simulink model "control_UAV"  (R2026a)
settings: Solver=VariableStepAuto  StopTime=30
values from neighbouring files (symbols this model uses):
  b = P.rotor.b    [Inicializacion.m]
  chen_a = 35    [Inicializacion.m]
  chen_b = 3    [Inicializacion.m]
  chen_c = 28    [Inicializacion.m]
  chen_center_z = 30    [Inicializacion.m]
  chen_scale_x = 30    [Inicializacion.m]
  chen_scale_y = 35    [Inicializacion.m]
  chen_scale_z = 30    [Inicializacion.m]
  d = P.rotor.d    [Inicializacion.m]
  g = P.g    [Inicializacion.m]
  Jr = P.Jr    [Inicializacion.m]
  Jxx = P.Jxx    [Inicializacion.m]
  Jyy = P.Jyy    [Inicializacion.m]
  Jzz = P.Jzz    [Inicializacion.m]
  kdphi = K.phi.Kd    [Inicializacion.m]
  kdpsi = K.psi.Kd    [Inicializacion.m]
  kdtheta = K.theta.Kd    [Inicializacion.m]
  kDx = P.aero.kDx    [Inicializacion.m]
  kdx = K.x.Kd    [Inicializacion.m]
  kDy = P.aero.kDy    [Inicializacion.m]
  kdy = K.y.Kd    [Inicializacion.m]
  kDz = P.aero.kDz    [Inicializacion.m]
  kdz = K.zAccel.Kd    [Inicializacion.m]
  kfax = P.kfax    [Inicializacion.m]
  kfay = P.kfay    [Inicializacion.m]
  kfaz = P.kfaz    [Inicializacion.m]
  kftx = P.kftx    [Inicializacion.m]
  kfty = P.kfty    [Inicializacion.m]
  kftz = P.kftz    [Inicializacion.m]
  kiphi = K.phi.Ki    [Inicializacion.m]
  kipsi = K.psi.Ki    [Inicializacion.m]
  kitheta = K.theta.Ki    [Inicializacion.m]
  kix = K.x.Ki    [Inicializacion.m]
  kiy = K.y.Ki    [Inicializacion.m]
  kiz = K.zAccel.Ki    [Inicializacion.m]
  kpphi = K.phi.Kp    [Inicializacion.m]
  kppsi = K.psi.Kp    [Inicializacion.m]
  kptheta = K.theta.Kp    [Inicializacion.m]
  kpx = K.x.Kp    [Inicializacion.m]
  kpy = K.y.Kp    [Inicializacion.m]
  kpz = K.zAccel.Kp    [Inicializacion.m]
  l = P.armLength    [Inicializacion.m]
  m = P.mass    [Inicializacion.m]
  omega_max = P.rotor.omegaMax    [Inicializacion.m]
  tau_motor = 0.05    [Inicializacion.m]
  Thover = K.Thover    [Inicializacion.m]
  Vw_max = P.aero.windSpeedMax    [Inicializacion.m]
undefined symbols (not defined in the file or in its folder): magnitude
settings Model: Creator=d1vad_l3gna  LastModifiedBy=D1vad L3gna

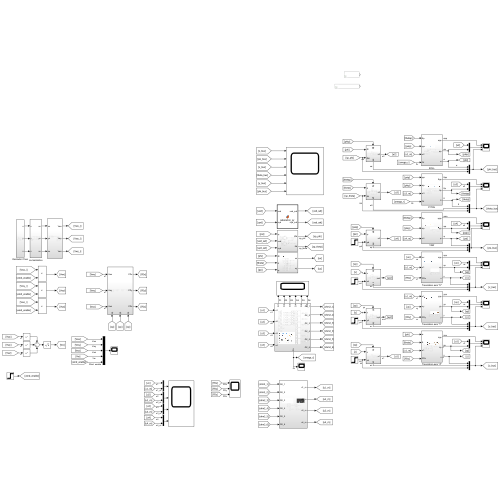
[thumbnail: Simulink's stored preview of the top-level diagram]
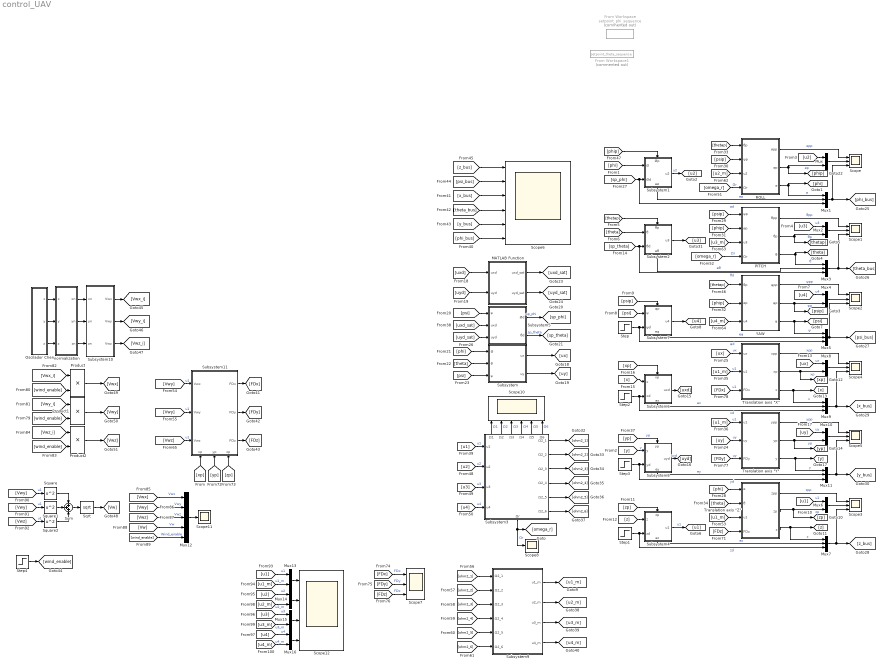
== system control_UAV ==
  From Workspace : FromWorkspace  Commented=on  VariableName=setpoint_phi_sequence  Interpolate=off  OutputAfterFinalValue=Holding final value
  From Workspace1 : FromWorkspace  Commented=on  VariableName=setpoint_theta_sequence  Interpolate=off  OutputAfterFinalValue=Holding final value
  MATLAB Function : MATLAB Function  TreatAsAtomicUnit=on
  Mux{,2,4,6,8,10,13..16} (10 alike) : Mux  Inputs=2
  Mux{1,3,5,7,9,11} (6 alike) : Mux  Inputs=3
  Mux12 : Mux  Inputs=5
  Oscilador Chen : Subsystem
  PITCH : Subsystem
  Product : Product
  Product1 : Product
  Product2 : Product
  ROLL : Subsystem
  Scope{,1..5,7} (7 alike) : Scope  NumInputPorts=3
      Scope settings: ActiveDisplayYMinimum=-134.04297196202708  ActiveDisplayYMaximum=108.05186605238116
      Scope1 settings: ActiveDisplayYMinimum=-2.6964368971416346  ActiveDisplayYMaximum=2.3091901291988428
      Scope2 settings: ActiveDisplayYMinimum=-20.085778959266992  ActiveDisplayYMaximum=163.07055659378912  DataLoggingVariableName=ScopeData2
      Scope3 settings: ActiveDisplayYMinimum=-60.018912358895363  ActiveDisplayYMaximum=169.44654581765505  DataLoggingVariableName=ScopeData3
      Scope4 settings: ActiveDisplayYMinimum=-60.018912358895363  ActiveDisplayYMaximum=169.44654581765505  DataLoggingVariableName=ScopeData4
      Scope5 settings: ActiveDisplayYMinimum=-4.0823822518726  ActiveDisplayYMaximum=2.5647555738372825  DataLoggingVariableName=ScopeData5
      Scope7 settings: ActiveDisplayString=3  ActiveDisplayYMinimum=-1.1101406632308159  ActiveDisplayYMaximum=0.27802164773982191  DataLoggingVariableName=ScopeData7
  Scope10 : Scope  NumInputPorts=6
      settings: ActiveDisplayYMinimum=-90.652821559527951  ActiveDisplayYMaximum=815.8753940357517  DataLoggingVariableName=ScopeData10
  Scope11 : Scope
      settings: ActiveDisplayYMinimum=-7.1247044664866621  ActiveDisplayYMaximum=8.6160020821192056  DataLoggingVariableName=ScopeData11
  Scope12 : Scope  NumInputPorts=4
      settings: ActiveDisplayYMinimum=-56.813279862399021  ActiveDisplayYMaximum=511.31951876159133  DataLoggingVariableName=ScopeData12
  Scope6 : Scope  NumInputPorts=6
      settings: ActiveDisplayYMinimum=-0.7400477310754251  ActiveDisplayYMaximum=5.6591974559880578  DataLoggingVariableName=ScopeData6
  Scope8 : Scope
      settings: ActiveDisplayYMinimum=-4.4408920985006262E-15  ActiveDisplayYMaximum=4.4408920985006262E-15  DataLoggingVariableName=ScopeData8
  Sqrt : Sqrt
  Square : Math  Operator=square
  Square1 : Math  Operator=square
  Square2 : Math  Operator=square
  Step : Step  Time=0  FinalValue=0  SampleTime=0
  Step1 : Step  FinalValue=5  SampleTime=0
  Step2 : Step  Time=4  FinalValue=5  SampleTime=0
  Step3 : Step  Time=0  FinalValue=0  SampleTime=0
  Step4 : Step  Time=9  SampleTime=0
  Subsystem : Subsystem
  Subsystem1 : Subsystem
      settings: PortSchema="{\"entries\":[{\"content\":{\"sides\":[{\"content\":{\"connectorIds\":[\"In1\",\"In2\"]},\"type\":\"ConnectorPlacement.EquallySpacedRectSide\",\"uuid\":\"d3a3a6fe-31b6-42e8-8951-59acef78037d\"},{\"content\":{\"connectorIds\":[\"Out1\"],\"side\":\"RIGHT\"},\"type\":\"ConnectorPlacement.EquallySpacedRectSide\",\"uuid\":\"98a273af-9231-4eb5-99d8-49a6c653f3f8\"},{\"content\":{\"connectorIds\":[\"In3\"],\"side\":\"TOP\"},\"type\":\"ConnectorPlacement.EquallySpacedRectSide\",\"uuid\":\"3e4d54af-1b05-4072-bd7d-c924a9f6a300\"},{\"content\":{\"connectorIds\":[\"Out2\"],\"side\":\"BOTTOM\"},\"type\":\"ConnectorPlacement.EquallySpacedRectSide\",\"uuid\":\"dbda693a-fe86-48a0-894d-0bd0198370e6\"}]},\"type\":\"ConnectorPlacement.EquallySpacedConnector\",\"uuid\":\"caea40f7-b591-4aba-8407-638933b38774\"}],\"packageUris\":[\"http://schema.mathworks.com/mf0/Connector/R2020b\"],\"version\":\"1.0\"}"
  Subsystem10 : Subsystem
  Subsystem11 : Subsystem
      settings: PortSchema="{\"entries\":[{\"content\":{\"sides\":[{\"content\":{\"connectorIds\":[\"In1\",\"In2\",\"In3\"]},\"type\":\"ConnectorPlacement.EquallySpacedRectSide\",\"uuid\":\"354ce72d-1d6c-4cc8-9e91-463c07f034cd\"},{\"content\":{\"connectorIds\":[\"Out1\",\"Out2\",\"Out3\"],\"side\":\"RIGHT\"},\"type\":\"ConnectorPlacement.EquallySpacedRectSide\",\"uuid\":\"d4bbd9c4-471b-4074-a3af-0e8a4cf51752\"},{\"content\":{\"side\":\"TOP\"},\"type\":\"ConnectorPlacement.EquallySpacedRectSide\",\"uuid\":\"5e614824-097c-4c07-9e45-0c4f9bbdd2e4\"},{\"content\":{\"connectorIds\":[\"In4\",\"In5\",\"In6\"],\"side\":\"BOTTOM\"},\"type\":\"ConnectorPlacement.EquallySpacedRectSide\",\"uuid\":\"b8e7f3a6-70ea-469a-9568-8fe2ed1a39af\"}]},\"type\":\"ConnectorPlacement.EquallySpacedConnector\",\"uuid\":\"e757125c-b99d-4f23-b824-7aca730001ba\"}],\"packageUris\":[\"http://schema.mathworks.com/mf0/Connector/R2020b\"],\"version\":\"1.0\"}"
  Subsystem2 : Subsystem
      settings: PortSchema="{\"entries\":[{\"content\":{\"sides\":[{\"content\":{\"connectorIds\":[\"In1\",\"In2\"]},\"type\":\"ConnectorPlacement.EquallySpacedRectSide\",\"uuid\":\"c42bea5d-3df1-43f4-8461-fc0f8e0dbc4c\"},{\"content\":{\"connectorIds\":[\"Out1\"],\"side\":\"RIGHT\"},\"type\":\"ConnectorPlacement.EquallySpacedRectSide\",\"uuid\":\"72025c3e-c054-42d9-8613-22244a708765\"},{\"content\":{\"connectorIds\":[\"In3\"],\"side\":\"TOP\"},\"type\":\"ConnectorPlacement.EquallySpacedRectSide\",\"uuid\":\"4b6680ac-412c-41ad-b127-e39dee57a48b\"},{\"content\":{\"connectorIds\":[\"Out2\"],\"side\":\"BOTTOM\"},\"type\":\"ConnectorPlacement.EquallySpacedRectSide\",\"uuid\":\"172eadf6-2acd-43c4-907f-43e59ecf9406\"}]},\"type\":\"ConnectorPlacement.EquallySpacedConnector\",\"uuid\":\"ee6badca-de14-4676-af90-b761200effe4\"}],\"packageUris\":[\"http://schema.mathworks.com/mf0/Connector/R2020b\"],\"version\":\"1.0\"}"
  Subsystem3 : Subsystem
      settings: PortSchema="{\"entries\":[{\"content\":{\"sides\":[{\"content\":{\"connectorIds\":[\"In1\",\"In2\",\"In3\",\"In4\"]},\"type\":\"ConnectorPlacement.EquallySpacedRectSide\",\"uuid\":\"bbf73f2c-001a-4d28-bdc9-6d66d68f2ea4\"},{\"content\":{\"connectorIds\":[\"Out1\",\"Out2\",\"Out3\",\"Out4\",\"Out5\",\"Out6\"],\"side\":\"RIGHT\"},\"type\":\"ConnectorPlacement.EquallySpacedRectSide\",\"uuid\":\"2f04f957-8e88-4bc3-9b02-53fc0fb1d7f8\"},{\"content\":{\"connectorIds\":[\"Out8\",\"Out9\",\"Out10\",\"Out11\",\"Out12\",\"Out13\"],\"side\":\"TOP\"},\"type\":\"ConnectorPlacement.EquallySpacedRectSide\",\"uuid\":\"66771ef2-ad1a-4f4f-bfbc-325ca576d4d7\"},{\"content\":{\"connectorIds\":[\"Out7\"],\"side\":\"BOTTOM\"},\"type\":\"ConnectorPlacement.EquallySpacedRectSide\",\"uuid\":\"4f342048-b513-46d4-854a-b011df012f9d\"}]},\"type\":\"ConnectorPlacement.EquallySpacedConnector\",\"uuid\":\"5b7006c4-ee2f-4b2d-a5a4-3391366b57a8\"}],\"packageUris\":[\"http://schema.mathworks.com/mf0/Connector/R2020b\"],\"version\":\"1.0\"}"
  Subsystem4 : Subsystem
      settings: PortSchema="{\"entries\":[{\"content\":{\"sides\":[{\"content\":{\"connectorIds\":[\"In1\",\"In2\"]},\"type\":\"ConnectorPlacement.EquallySpacedRectSide\",\"uuid\":\"05b9bfb1-b25d-4f19-883a-8c73fb6ccdf1\"},{\"content\":{\"connectorIds\":[\"Out1\"],\"side\":\"RIGHT\"},\"type\":\"ConnectorPlacement.EquallySpacedRectSide\",\"uuid\":\"b5ec7534-1bb3-4079-b442-bebab7b7e6ff\"},{\"content\":{\"connectorIds\":[\"In3\"],\"side\":\"TOP\"},\"type\":\"ConnectorPlacement.EquallySpacedRectSide\",\"uuid\":\"45979954-0dce-4b5e-a8a1-be246f039e3e\"},{\"content\":{\"connectorIds\":[\"Out2\"],\"side\":\"BOTTOM\"},\"type\":\"ConnectorPlacement.EquallySpacedRectSide\",\"uuid\":\"2779124c-2f03-4275-9de9-8b69c4e3182f\"}]},\"type\":\"ConnectorPlacement.EquallySpacedConnector\",\"uuid\":\"2b80c90b-fdf2-4625-bada-2e722c12cb75\"}],\"packageUris\":[\"http://schema.mathworks.com/mf0/Connector/R2020b\"],\"version\":\"1.0\"}"
  Subsystem5 : Subsystem
  Subsystem6 : Subsystem
      settings: PortSchema="{\"entries\":[{\"content\":{\"sides\":[{\"content\":{\"connectorIds\":[\"In1\",\"In2\"]},\"type\":\"ConnectorPlacement.EquallySpacedRectSide\",\"uuid\":\"d3a3a6fe-31b6-42e8-8951-59acef78037d\"},{\"content\":{\"connectorIds\":[\"Out1\"],\"side\":\"RIGHT\"},\"type\":\"ConnectorPlacement.EquallySpacedRectSide\",\"uuid\":\"98a273af-9231-4eb5-99d8-49a6c653f3f8\"},{\"content\":{\"connectorIds\":[\"In3\"],\"side\":\"TOP\"},\"type\":\"ConnectorPlacement.EquallySpacedRectSide\",\"uuid\":\"3e4d54af-1b05-4072-bd7d-c924a9f6a300\"},{\"content\":{\"connectorIds\":[\"Out2\"],\"side\":\"BOTTOM\"},\"type\":\"ConnectorPlacement.EquallySpacedRectSide\",\"uuid\":\"04a05dfd-3838-43e0-9a0f-9dddf1e0efcf\"}]},\"type\":\"ConnectorPlacement.EquallySpacedConnector\",\"uuid\":\"caea40f7-b591-4aba-8407-638933b38774\"}],\"packageUris\":[\"http://schema.mathworks.com/mf0/Connector/R2020b\"],\"version\":\"1.0\"}"
  Subsystem7 : Subsystem
      settings: PortSchema="{\"entries\":[{\"content\":{\"sides\":[{\"content\":{\"connectorIds\":[\"In1\",\"In2\"]},\"type\":\"ConnectorPlacement.EquallySpacedRectSide\",\"uuid\":\"75bf6914-bd39-4ffb-9926-3e582ee76d2e\"},{\"content\":{\"connectorIds\":[\"Out1\"],\"side\":\"RIGHT\"},\"type\":\"ConnectorPlacement.EquallySpacedRectSide\",\"uuid\":\"c513c889-9702-4896-9634-182684fb2270\"},{\"content\":{\"connectorIds\":[\"In3\"],\"side\":\"TOP\"},\"type\":\"ConnectorPlacement.EquallySpacedRectSide\",\"uuid\":\"615aeb91-fdc7-410e-8ef1-be935f8f6065\"},{\"content\":{\"connectorIds\":[\"Out2\"],\"side\":\"BOTTOM\"},\"type\":\"ConnectorPlacement.EquallySpacedRectSide\",\"uuid\":\"e306c6e8-76f5-43f1-b56c-f57f2096c31d\"}]},\"type\":\"ConnectorPlacement.EquallySpacedConnector\",\"uuid\":\"5b277172-4ad9-4051-981d-00b9cba435ce\"}],\"packageUris\":[\"http://schema.mathworks.com/mf0/Connector/R2020b\"],\"version\":\"1.0\"}"
  Subsystem8 : Subsystem
      settings: PortSchema="{\"entries\":[{\"content\":{\"sides\":[{\"content\":{\"connectorIds\":[\"In1\",\"In2\"]},\"type\":\"ConnectorPlacement.EquallySpacedRectSide\",\"uuid\":\"d3a3a6fe-31b6-42e8-8951-59acef78037d\"},{\"content\":{\"connectorIds\":[\"Out1\"],\"side\":\"RIGHT\"},\"type\":\"ConnectorPlacement.EquallySpacedRectSide\",\"uuid\":\"98a273af-9231-4eb5-99d8-49a6c653f3f8\"},{\"content\":{\"connectorIds\":[\"In3\"],\"side\":\"TOP\"},\"type\":\"ConnectorPlacement.EquallySpacedRectSide\",\"uuid\":\"3e4d54af-1b05-4072-bd7d-c924a9f6a300\"},{\"content\":{\"connectorIds\":[\"Out2\"],\"side\":\"BOTTOM\"},\"type\":\"ConnectorPlacement.EquallySpacedRectSide\",\"uuid\":\"3f53bca7-61ef-434d-b07d-c6d7aec8d75b\"}]},\"type\":\"ConnectorPlacement.EquallySpacedConnector\",\"uuid\":\"caea40f7-b591-4aba-8407-638933b38774\"}],\"packageUris\":[\"http://schema.mathworks.com/mf0/Connector/R2020b\"],\"version\":\"1.0\"}"
  Subsystem9 : Subsystem
  Sum : Sum  Inputs=+++
  "Translation axis \"X\"" : Subsystem
  "Translation axis \"Y\"" : Subsystem
  "Translation axis \"Z\"" : Subsystem
  YAW : Subsystem
  normalization : Subsystem
  wires:
  Subsystem1/1(u2) -> [u2]  "u2"
  [sp_phi] -> Mux1/3, Subsystem1/2(Ød)  "ød"
  Mux1/1 -> [phi_bus], Scope/3
  Mux/1 -> Scope/2
  [phi] -> Subsystem1/1(Ø)
  ROLL/1(øpp) -> Scope/1  "øpp"
  ROLL/2(øp) -> Mux/2, [phip]  "øp"
  ROLL/3(ø) -> [phi], Mux1/1  "ø"
  Subsystem1/2(eø) -> Mux1/2  "eø"
  Mux2/1 -> Scope1/2
  [sp_theta] -> Mux3/3, Subsystem2/2(θd)  "θd"
  PITCH/3(θ) -> [theta], Mux3/1  "θ"
  Subsystem2/2(eθ) -> Mux3/2  "eθ"
  Mux3/1 -> Scope1/3, [theta_bus]
  [thetap] -> Subsystem2/3(θp)
  PITCH/2(θp) -> Mux2/2, [thetap]  "θp"
  PITCH/1(θpp) -> Scope1/1  "θpp"
  [thetap] -> YAW/1(θp)
  YAW/1(ψpp) -> Scope2/1  "ψpp"
  YAW/2(ψp) -> [psip], Mux4/2  "ψp"
  Subsystem7/1(u4) -> [u4]
  Step/1 -> Mux5/3, Subsystem7/2(ψd)  "ψd"
  [u4] -> Mux4/1  "u4"
  Mux4/1 -> Scope2/2
  Mux5/1 -> Scope2/3, [psi_bus]
  YAW/3(ψ) -> Mux5/1, [psi]  "ψ"
  [psi] -> Subsystem7/1(ψ)
  [psip] -> Subsystem7/3(ψp)
  Subsystem7/2(eψ) -> Mux5/2  "eψ"
  [phi] -> "Translation axis \"Z\""/1(ø)
  [theta] -> "Translation axis \"Z\""/2(θ)
  Subsystem4/1(u1) -> [u1]  "u1"
  [u1] -> Mux6/1  "u1"
  "Translation axis \"Z\""/2(zp) -> [zp], Mux6/2  "zp"
  Step1/1 -> Mux7/3, Subsystem4/2(zd)  "zd"
  "Translation axis \"Z\""/3(z) -> Mux7/1, [z]  "z"
  Subsystem4/2(ez) -> Mux7/2  "ez"
  [zp] -> Subsystem4/3(zp)
  [z] -> Subsystem4/1(z)
  Mux6/1 -> Scope3/2
  Mux7/1 -> [z_bus], Scope3/3
  "Translation axis \"Z\""/1(zpp) -> Scope3/1  "zpp"
  Step2/1 -> Mux9/3, Subsystem6/2(xd)  "xd"
  [ux] -> Mux8/1  "ux"
  Mux8/1 -> Scope4/2
  "Translation axis \"X\""/1(xpp) -> Scope4/1  "xpp"
  "Translation axis \"X\""/2(xp) -> [xp], Mux8/2  "xp"
  "Translation axis \"X\""/3(x) -> Mux9/1, [x]  "x"
  [xp] -> Subsystem6/3(xp)
  [x] -> Subsystem6/1(x)
  Subsystem6/2(ex) -> Mux9/2  "ex"
  Mux9/1 -> [x_bus], Scope4/3
  Subsystem6/1(uxd) -> [uxd]
  Subsystem8/1(uyd) -> [uyd]  "uyd"
  Step3/1 -> Mux11/3, Subsystem8/2(yd)  "yd"
  Mux10/1 -> Scope5/2
  "Translation axis \"Y\""/1(ypp) -> Scope5/1  "ypp"
  [uy] -> Mux10/1  "uy"
  "Translation axis \"Y\""/2(yp) -> Mux10/2, [yp]  "yp"
  "Translation axis \"Y\""/3(y) -> Mux11/1, [y]  "y"
  Mux11/1 -> [y_bus], Scope5/3
  Subsystem8/2(ey) -> Mux11/2  "ey"
  [phi] -> Subsystem/1(Ø)
  [theta] -> Subsystem/2(θ)
  [psi] -> Subsystem/3(ψ)
  Subsystem/1(ux) -> [ux]
  Subsystem/2(uy) -> [uy]
  [uy] -> "Translation axis \"Y\""/2(uy)  "uy"
  [ux] -> "Translation axis \"X\""/1(ux)  "ux"
  Subsystem5/1(Ød) -> [sp_phi]  "sp_phi"
  Subsystem5/2(θd) -> [sp_theta]  "sp_theta"
  [u1_m] -> "Translation axis \"X\""/2(u1)  "u1"
  [u1_m] -> "Translation axis \"Y\""/1(u1)  "u1"
  [psi] -> Subsystem5/1(ψ)
  [uxd] -> MATLAB Function/1(uxd)
  [uyd] -> MATLAB Function/2(uyd)
  MATLAB Function/1(uxd_sat) -> [uxd_sat]
  MATLAB Function/2(uyd_sat) -> [uyd_sat]
  [uxd_sat] -> Subsystem5/2(uxd)
  [uyd_sat] -> Subsystem5/3(uyd)
  [z_bus] -> Scope6/1
  [psi_bus] -> Scope6/2
  [x_bus] -> Scope6/3
  [theta_bus] -> Scope6/4
  [y_bus] -> Scope6/5
  [phi_bus] -> Scope6/6
  [thetap] -> ROLL/1(θp)
  [psip] -> PITCH/1(ψp)
  [phip] -> PITCH/2(øp)
  [phip] -> YAW/2(øp)
  [yp] -> Subsystem8/3(yp)  "yp"
  [y] -> Subsystem8/1(y)  "y"
  [phip] -> Subsystem1/3(Øp)
  [theta] -> Subsystem2/1(θ)
  [u2] -> Mux/1
  [u3] -> Mux2/1  "u3"
  Subsystem2/1(u3) -> [u3]
  [psip] -> ROLL/2(ψp)
  [u1] -> Subsystem3/1(u1)  "u1"
  [u2] -> Subsystem3/2(u2)  "u2"
  [u3] -> Subsystem3/3(u3)  "u3"
  [u4] -> Subsystem3/4(u4)  "u4"
  Subsystem3/7(Ωr) -> [omega_r], Scope8/1  "Ωr"
  [omega_r] -> ROLL/4(Ωr)  "Ωr"
  [omega_r] -> PITCH/4(Ωr)  "Ωr"
  [u1_m] -> "Translation axis \"Z\""/3(u1)
  Subsystem3/2(Ω2_2) -> [ohm2_2]
  Subsystem3/3(Ω2_3) -> [ohm2_3]
  Subsystem3/4(Ω2_4) -> [ohm2_4]
  Subsystem3/6(Ω2_6) -> [ohm2_6]
  Subsystem3/8(Ω1) -> Scope10/1  "Ω1"
  Subsystem3/9(Ω2) -> Scope10/2  "Ω2"
  Subsystem3/10(Ω3) -> Scope10/3  "Ω3"
  Subsystem3/11(Ω4) -> Scope10/4  "Ω4"
  Subsystem3/12(Ω5) -> Scope10/5  "Ω5"
  Subsystem3/13(Ω6) -> Scope10/6  "Ω6"
  [ohm2_1] -> Subsystem9/1(Ω2_1)
  [ohm2_2] -> Subsystem9/2(Ω2_2)
  [ohm2_3] -> Subsystem9/3(Ω2_3)
  [ohm2_4] -> Subsystem9/4(Ω2_4)
  [ohm2_5] -> Subsystem9/5(Ω2_5)
  [ohm2_6] -> Subsystem9/6(Ω2_6)
  Subsystem9/1(u1_m) -> [u1_m]
  Subsystem9/2(u2_m) -> [u2_m]
  Subsystem9/3(u3_m) -> [u3_m]
  Subsystem9/4(u4_m) -> [u4_m]
  [u2_m] -> ROLL/3(u2)
  [u3_m] -> PITCH/3(u3)
  [u4_m] -> YAW/3(u4)
  Subsystem3/1(Ω2_1) -> [ohm2_1]
  Subsystem3/5(Ω2_5) -> [ohm2_5]
  Oscilador Chen/1(x) -> normalization/1(x)
  Oscilador Chen/2(y) -> normalization/2(y)
  Oscilador Chen/3(z) -> normalization/3(z)
  normalization/1(xn) -> Subsystem10/1(xn)
  normalization/2(yn) -> Subsystem10/2(yn)
  normalization/3(zn) -> Subsystem10/3(zn)
  [FDz] -> "Translation axis \"Z\""/4(FDz)
  [xp] -> Subsystem11/4(xp)
  [yp] -> Subsystem11/5(yp)
  [zp] -> Subsystem11/6(zp)
  Subsystem11/1(FDx) -> [FDx]
  Subsystem11/2(FDy) -> [FDy]
  Subsystem11/3(FDz) -> [FDz]
  [FDx] -> Scope7/1  "FDx"
  [FDy] -> Scope7/2  "FDy"
  [FDz] -> Scope7/3  "FDz"
  [FDy] -> "Translation axis \"Y\""/3(FDy)  "uy"
  [FDx] -> "Translation axis \"X\""/3(FDx)  "u1"
  Step4/1 -> [wind_enable]
  [wind_enable] -> Product/2
  Subsystem10/1(Vwx) -> [Vwx_i]
  Subsystem10/2(Vwy) -> [Vwy_i]
  Subsystem10/3(Vwz) -> [Vwz_i]
  [Vwx_i] -> Product/1
  [Vwy_i] -> Product1/1
  [wind_enable] -> Product1/2
  [wind_enable] -> Product2/2
  [Vwz_i] -> Product2/1
  Mux12/1 -> Scope11/1
  [Vwx] -> Mux12/1  "Vwx"
  [Vwy] -> Mux12/2  "Vwy"
  [Vwz] -> Mux12/3  "Vwz"
  [Vw] -> Mux12/4  "Vw"
  [wind_enable] -> Mux12/5  "Wind_enable"
  [Vwy] -> Square/1  "u1"
  Square/1 -> Sum/1
  Square1/1 -> Sum/2
  Square2/1 -> Sum/3
  Sum/1 -> Sqrt/1
  [Vwy] -> Square1/1  "u1"
  [Vwz] -> Square2/1  "u1"
  Sqrt/1 -> [Vw]
  Mux13/1 -> Scope12/1
  [u1] -> Mux13/1  "u1"
  [u1_m] -> Mux13/2  "u1_m"
  Mux14/1 -> Scope12/2
  Mux15/1 -> Scope12/3
  Mux16/1 -> Scope12/4
  [u2] -> Mux14/1  "u2"
  [u3] -> Mux15/1  "u3"
  [u4] -> Mux16/1  "u4"
  [u2_m] -> Mux14/2  "u2_m"
  [u3_m] -> Mux15/2  "u3_m"
  [u4_m] -> Mux16/2  "u4_m"
  Product/1 -> [Vwx]
  Product1/1 -> [Vwy]
  Product2/1 -> [Vwz]
  [Vwy] -> Subsystem11/1(Vwx)  "u1"
  [Vwy] -> Subsystem11/2(Vwy)  "u1"
  [Vwz] -> Subsystem11/3(Vwz)  "u1"

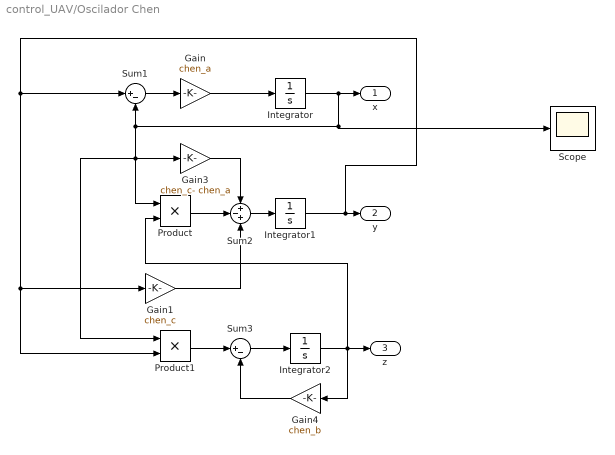
== system control_UAV/Oscilador Chen ==
  Gain : Gain  Gain=chen_a
  Gain1 : Gain  Gain=chen_c
  Gain3 : Gain  Gain=chen_c- chen_a
  Gain4 : Gain  Gain=chen_b
  Integrator : Integrator
  Integrator1 : Integrator  InitialCondition=0.1
  Integrator2 : Integrator
  Product : Product
  Product1 : Product
  Scope : Scope
      settings: ActiveDisplayYMinimum=-1  ActiveDisplayYMaximum=1  DataLoggingVariableName=ScopeData2
  Sum1 : Sum  Inputs=|+-
  Sum2 : Sum  Inputs=+-+
  Sum3 : Sum  Inputs=|+-
  x : Outport
  y : Outport  Port=2
  z : Outport  Port=3
  wires:
  Sum1/1 -> Gain/1
  Gain/1 -> Integrator/1
  Integrator1/1 -> Sum1/1, Gain1/1, Product1/2, y/1
  Gain3/1 -> Sum2/1
  Sum2/1 -> Integrator1/1
  Integrator2/1 -> Product/2, Gain4/1, z/1
  Product/1 -> Sum2/2
  Gain1/1 -> Sum2/3
  Integrator/1 -> Scope/1, Product1/1, Product/1, Gain3/1, Sum1/2, x/1
  Product1/1 -> Sum3/1
  Sum3/1 -> Integrator2/1
  Gain4/1 -> Sum3/2

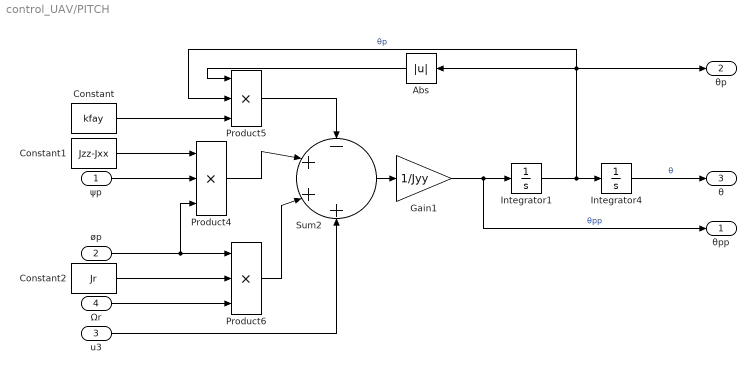
== system control_UAV/PITCH ==
  ψp : Inport
  øp : Inport  Port=2
  u3 : Inport  Port=3
  Ωr : Inport  Port=4
  Abs : Abs  SaturateOnIntegerOverflow=off
  Constant : Constant  Value=kfay
  Constant1 : Constant  Value=Jzz-Jxx
  Constant2 : Constant  Value=Jr
  Gain1 : Gain  Gain=1/Jyy
  Integrator1 : Integrator
  Integrator4 : Integrator
  Product4 : Product  Inputs=3
  Product5 : Product  Inputs=3
  Product6 : Product  Inputs=3
  Sum2 : Sum  Inputs=-+++
  θpp : Outport
  θp : Outport  Port=2
  θ : Outport  Port=3
  wires:
  Abs/1 -> Product5/1
  u3/1 -> Sum2/4
  Product4/1 -> Sum2/2
  ψp/1 -> Product4/2
  Sum2/1 -> Gain1/1
  Product5/1 -> Sum2/1
  Constant/1 -> Product5/3
  Integrator4/1 -> θ/1  "θ"
  Gain1/1 -> Integrator1/1, θpp/1  "θpp"
  Constant2/1 -> Product6/2
  Product6/1 -> Sum2/3
  Constant1/1 -> Product4/1
  Integrator1/1 -> Integrator4/1, Product5/2, Abs/1, θp/1  "θp"
  øp/1 -> Product6/1, Product4/3
  Ωr/1 -> Product6/3

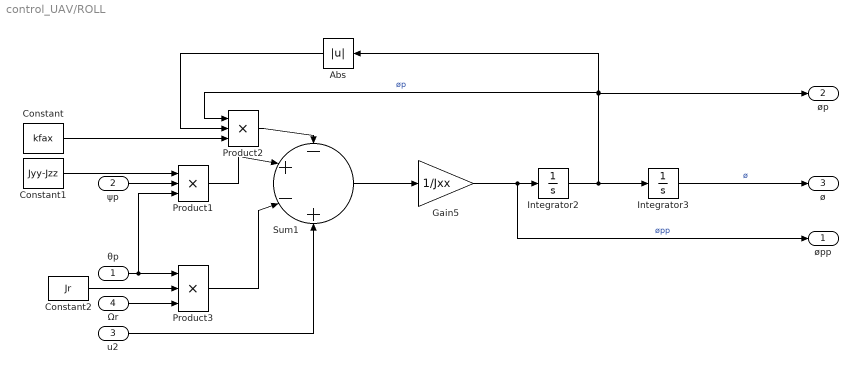
== system control_UAV/ROLL ==
  θp : Inport
  ψp : Inport  Port=2
  u2 : Inport  Port=3
  Ωr : Inport  Port=4
  Abs : Abs  SaturateOnIntegerOverflow=off
  Constant : Constant  Value=kfax
  Constant1 : Constant  Value=Jyy-Jzz
  Constant2 : Constant  Value=Jr
  Gain5 : Gain  Gain=1/Jxx
  Integrator2 : Integrator
  Integrator3 : Integrator
  Product1 : Product  Inputs=3
  Product2 : Product  Inputs=3
  Product3 : Product  Inputs=3
  Sum1 : Sum  Inputs=-+-+
  øpp : Outport
  øp : Outport  Port=2
  ø : Outport  Port=3
  wires:
  Product3/1 -> Sum1/3
  θp/1 -> Product1/3, Product3/1
  Integrator2/1 -> Product2/1, Abs/1, øp/1, Integrator3/1  "øp"
  Gain5/1 -> øpp/1, Integrator2/1  "øpp"
  Sum1/1 -> Gain5/1
  Product1/1 -> Sum1/2
  Constant1/1 -> Product1/1
  Integrator3/1 -> ø/1  "ø"
  u2/1 -> Sum1/4
  ψp/1 -> Product1/2
  Product2/1 -> Sum1/1
  Constant/1 -> Product2/3
  Abs/1 -> Product2/2
  Ωr/1 -> Product3/3
  Constant2/1 -> Product3/2

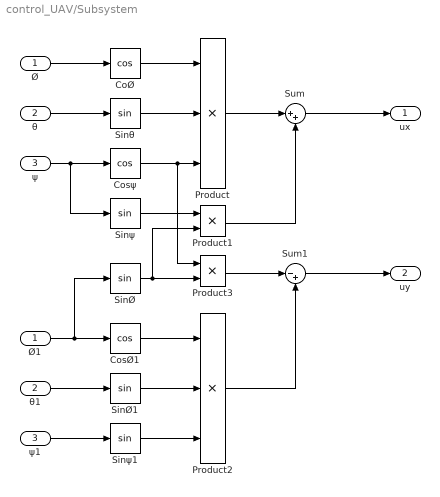
== system control_UAV/Subsystem ==
  Ø : Inport
  θ : Inport  Port=2
  ψ : Inport  Port=3
  CosØ1 : Trigonometry  Operator=cos
  Cosψ : Trigonometry  Operator=cos
  CoØ : Trigonometry  Operator=cos
  Product : Product  Inputs=3
  Product1 : Product
  Product2 : Product  Inputs=3
  Product3 : Product
  SinØ : Trigonometry
  SinØ1 : Trigonometry
  Sinθ : Trigonometry
  Sinψ : Trigonometry
  Sinψ1 : Trigonometry
  Sum : Sum  Inputs=|++
  Sum1 : Sum  Inputs=|-+
  Ø1 : InportShadow
  θ1 : InportShadow  Port=2
  ψ1 : InportShadow  Port=3
  ux : Outport
  uy : Outport  Port=2
  wires:
  Ø/1 -> CoØ/1
  θ/1 -> Sinθ/1
  ψ/1 -> Sinψ/1, Cosψ/1
  CoØ/1 -> Product/1
  Sinθ/1 -> Product/2
  Cosψ/1 -> Product3/1, Product/3
  Product/1 -> Sum/1
  Product1/1 -> Sum/2
  Sum/1 -> ux/1
  Sinψ1/1 -> Product2/3
  SinØ1/1 -> Product2/2
  CosØ1/1 -> Product2/1
  ψ1/1 -> Sinψ1/1
  θ1/1 -> SinØ1/1
  Ø1/1 -> SinØ/1, CosØ1/1
  Sinψ/1 -> Product1/1
  SinØ/1 -> Product3/2, Product1/2
  Product2/1 -> Sum1/2
  Product3/1 -> Sum1/1
  Sum1/1 -> uy/1

== system control_UAV/Subsystem1 ==
  Ø : Inport
  Ød : Inport  Port=2
  Øp : Inport  Port=3
  Gain6 : Gain  Gain=kdphi
  Gain7 : Gain  Gain=kiphi
  Gain9 : Gain  Gain=kpphi
  Integrator1 : Integrator
  Sum2 : Sum  Inputs=|+-
  Sum3 : Sum  Inputs=++-
  u2 : Outport
  eø : Outport  Port=2
  wires:
  Sum2/1 -> eø/1, Gain9/1, Gain7/1
  Gain9/1 -> Sum3/1
  Ø/1 -> Sum2/2
  Integrator1/1 -> Sum3/2
  Ød/1 -> Sum2/1
  Gain6/1 -> Sum3/3
  Gain7/1 -> Integrator1/1
  Sum3/1 -> u2/1
  Øp/1 -> Gain6/1

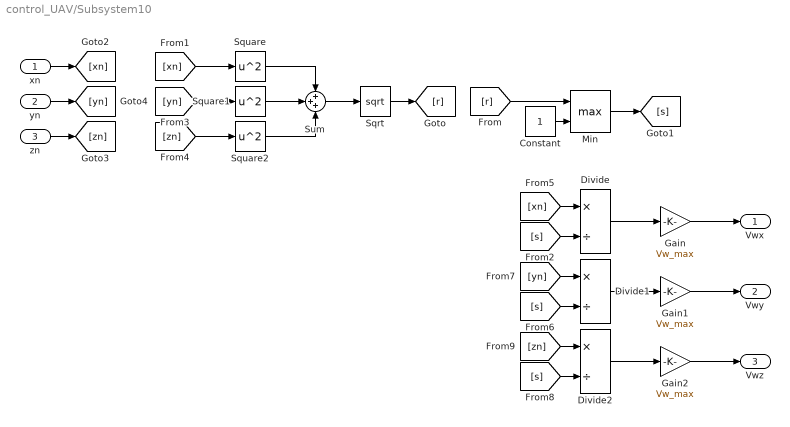
== system control_UAV/Subsystem10 ==
  xn : Inport
  yn : Inport  Port=2
  zn : Inport  Port=3
  Constant : Constant
  Divide : Product  Inputs=*/
  Divide1 : Product  Inputs=*/
  Divide2 : Product  Inputs=*/
  Gain : Gain  Gain=Vw_max
  Gain1 : Gain  Gain=Vw_max
  Gain2 : Gain  Gain=Vw_max
  Min : MinMax  Function=max  Inputs=2
  Sqrt : Sqrt
  Square : Math  Operator=square
  Square1 : Math  Operator=square
  Square2 : Math  Operator=square
  Sum : Sum  Inputs=+++
  Vwx : Outport
  Vwy : Outport  Port=2
  Vwz : Outport  Port=3
  wires:
  [xn] -> Square/1
  [yn] -> Square1/1
  [zn] -> Square2/1
  Square/1 -> Sum/1
  Square1/1 -> Sum/2
  Square2/1 -> Sum/3
  Sum/1 -> Sqrt/1
  [r] -> Min/1
  Constant/1 -> Min/2
  Sqrt/1 -> [r]
  Min/1 -> [s]
  [s] -> Divide/2
  xn/1 -> [xn]
  zn/1 -> [zn]
  yn/1 -> [yn]
  [xn] -> Divide/1
  [yn] -> Divide1/1
  [s] -> Divide1/2
  [s] -> Divide2/2
  [zn] -> Divide2/1
  Divide/1 -> Gain/1
  Divide1/1 -> Gain1/1
  Divide2/1 -> Gain2/1
  Gain/1 -> Vwx/1
  Gain1/1 -> Vwy/1
  Gain2/1 -> Vwz/1

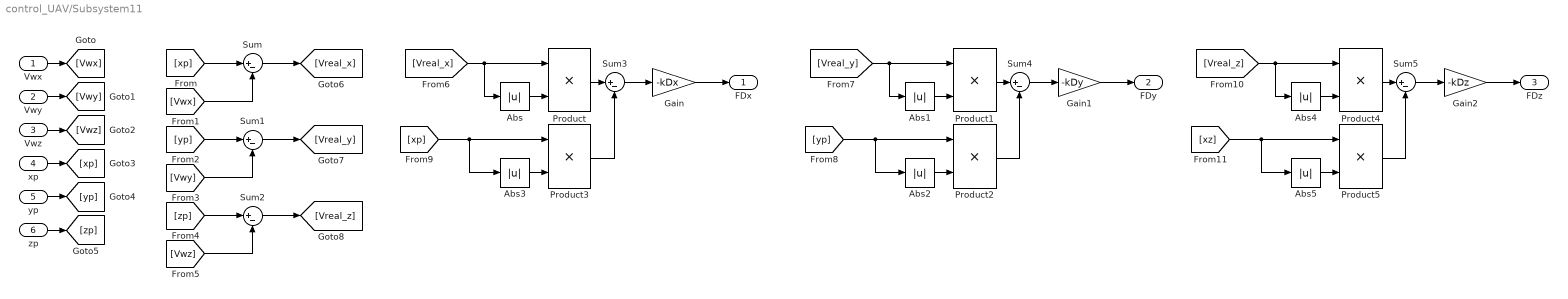
== system control_UAV/Subsystem11 ==
  Vwx : Inport
  Vwy : Inport  Port=2
  Vwz : Inport  Port=3
  xp : Inport  Port=4
  yp : Inport  Port=5
  zp : Inport  Port=6
  Abs{,1..5} (6 alike) : Abs  SaturateOnIntegerOverflow=off
  Gain : Gain  Gain=-kDx
  Gain1 : Gain  Gain=-kDy
  Gain2 : Gain  Gain=-kDz
  Product{,1..5} (6 alike) : Product
  Sum{,1..5} (6 alike) : Sum  Inputs=|+-
  FDx : Outport
  FDy : Outport  Port=2
  FDz : Outport  Port=3
  wires:
  Vwx/1 -> [Vwx]
  zp/1 -> [zp]
  Vwy/1 -> [Vwy]
  Vwz/1 -> [Vwz]
  xp/1 -> [xp]
  yp/1 -> [yp]
  [xp] -> Sum/1
  [Vwx] -> Sum/2
  Sum/1 -> [Vreal_x]
  Sum1/1 -> [Vreal_y]
  [Vwy] -> Sum1/2
  [yp] -> Sum1/1
  [zp] -> Sum2/1
  [Vwz] -> Sum2/2
  Sum2/1 -> [Vreal_z]
  [Vreal_x] -> Product/1, Abs/1
  Abs/1 -> Product/2
  Gain/1 -> FDx/1
  [xp] -> Abs3/1, Product3/1
  Abs3/1 -> Product3/2
  Product/1 -> Sum3/1
  Sum3/1 -> Gain/1
  Product3/1 -> Sum3/2
  Product2/1 -> Sum4/2
  Sum4/1 -> Gain1/1
  Product1/1 -> Sum4/1
  Abs2/1 -> Product2/2
  [yp] -> Product2/1, Abs2/1
  Gain1/1 -> FDy/1
  Abs1/1 -> Product1/2
  [Vreal_y] -> Abs1/1, Product1/1
  [Vreal_z] -> Product4/1, Abs4/1
  Abs4/1 -> Product4/2
  Gain2/1 -> FDz/1
  [xz] -> Abs5/1, Product5/1
  Abs5/1 -> Product5/2
  Product4/1 -> Sum5/1
  Sum5/1 -> Gain2/1
  Product5/1 -> Sum5/2

== system control_UAV/Subsystem2 ==
  θ : Inport
  θd : Inport  Port=2
  θp : Inport  Port=3
  Gain1 : Gain  Gain=kdtheta
  Gain11 : Gain  Gain=kitheta
  Gain12 : Gain  Gain=kptheta
  Integrator2 : Integrator
  Sum4 : Sum  Inputs=|+-
  Sum5 : Sum  Inputs=++-
  u3 : Outport
  eθ : Outport  Port=2
  wires:
  Sum4/1 -> Gain11/1, eθ/1, Gain12/1  "eθ"
  Gain12/1 -> Sum5/1
  θ/1 -> Sum4/2
  Integrator2/1 -> Sum5/2
  Gain11/1 -> Integrator2/1
  θd/1 -> Sum4/1
  Sum5/1 -> u3/1
  θp/1 -> Gain1/1
  Gain1/1 -> Sum5/3

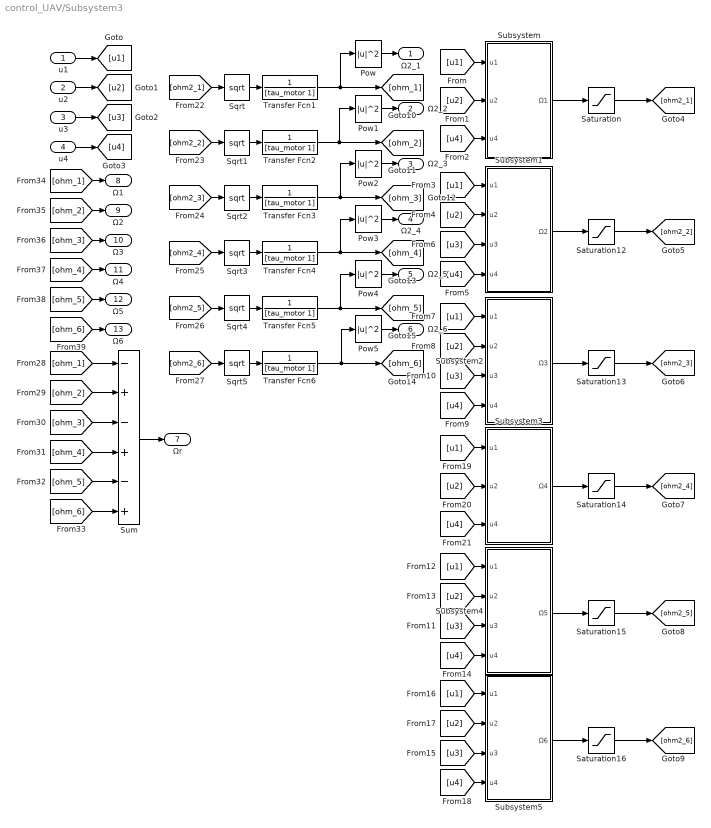
== system control_UAV/Subsystem3 ==
  u1 : Inport
  u2 : Inport  Port=2
  u3 : Inport  Port=3
  u4 : Inport  Port=4
  Pow{,1..5} (6 alike) : Math  Operator=magnitude^2  SignedPower=on  RndMeth=Zero
  Saturation{,12..16} (6 alike) : Saturate  UpperLimit=omega_max^2  LowerLimit=0
  Sqrt{,1..5} (6 alike) : Sqrt
  Subsystem : Subsystem
  Subsystem1 : Subsystem
  Subsystem2 : Subsystem
  Subsystem3 : Subsystem
  Subsystem4 : Subsystem
  Subsystem5 : Subsystem
  Sum : Sum  Inputs=-+-+-+
  Transfer Fcn{1..6} (6 alike) : TransferFcn  Denominator=[tau_motor 1]
  Ω2_1 : Outport
  Ω2_2 : Outport  Port=2
  Ω2_3 : Outport  Port=3
  Ω2_4 : Outport  Port=4
  Ω2_5 : Outport  Port=5
  Ω2_6 : Outport  Port=6
  Ωr : Outport  Port=7
  Ω1 : Outport  Port=8
  Ω2 : Outport  Port=9
  Ω3 : Outport  Port=10
  Ω4 : Outport  Port=11
  Ω5 : Outport  Port=12
  Ω6 : Outport  Port=13
  wires:
  Subsystem5/1(Ω6) -> Saturation16/1
  Subsystem4/1(Ω5) -> Saturation15/1
  Subsystem2/1(Ω3) -> Saturation13/1
  Subsystem3/1(Ω4) -> Saturation14/1
  Subsystem/1(Ω1) -> Saturation/1
  u1/1 -> [u1]
  u4/1 -> [u4]
  u3/1 -> [u3]
  u2/1 -> [u2]
  [u1] -> Subsystem/1(u1)
  [u2] -> Subsystem/2(u2)
  [u4] -> Subsystem/3(u4)
  [u1] -> Subsystem1/1(u1)
  [u2] -> Subsystem1/2(u2)
  [u4] -> Subsystem1/4(u4)
  [u3] -> Subsystem1/3(u3)
  Subsystem1/1(Ω2) -> Saturation12/1
  [u1] -> Subsystem2/1(u1)
  [u2] -> Subsystem2/2(u2)
  [u3] -> Subsystem2/3(u3)
  [u4] -> Subsystem2/4(u4)
  [u4] -> Subsystem4/4(u4)
  [u3] -> Subsystem4/3(u3)
  [u2] -> Subsystem4/2(u2)
  [u1] -> Subsystem4/1(u1)
  [u1] -> Subsystem5/1(u1)
  [u2] -> Subsystem5/2(u2)
  [u3] -> Subsystem5/3(u3)
  [u4] -> Subsystem5/4(u4)
  [u1] -> Subsystem3/1(u1)
  [u2] -> Subsystem3/2(u2)
  [u4] -> Subsystem3/3(u4)
  Sum/1 -> Ωr/1
  [ohm2_2] -> Sqrt1/1
  [ohm2_6] -> Sqrt5/1
  [ohm2_5] -> Sqrt4/1
  Sqrt2/1 -> Transfer Fcn3/1
  Sqrt1/1 -> Transfer Fcn2/1
  Sqrt4/1 -> Transfer Fcn5/1
  [ohm2_4] -> Sqrt3/1
  [ohm2_1] -> Sqrt/1
  Sqrt5/1 -> Transfer Fcn6/1
  Sqrt/1 -> Transfer Fcn1/1
  [ohm2_3] -> Sqrt2/1
  Sqrt3/1 -> Transfer Fcn4/1
  [ohm_1] -> Sum/1
  [ohm_3] -> Sum/3
  [ohm_4] -> Sum/4
  [ohm_5] -> Sum/5
  [ohm_6] -> Sum/6
  [ohm_2] -> Sum/2
  [ohm_2] -> Ω2/1
  [ohm_1] -> Ω1/1
  [ohm_6] -> Ω6/1
  [ohm_5] -> Ω5/1
  [ohm_4] -> Ω4/1
  [ohm_3] -> Ω3/1
  Transfer Fcn1/1 -> Pow/1, [ohm_1]
  Transfer Fcn2/1 -> Pow1/1, [ohm_2]
  Transfer Fcn3/1 -> Pow2/1, [ohm_3]
  Transfer Fcn4/1 -> Pow3/1, [ohm_4]
  Transfer Fcn5/1 -> Pow4/1, [ohm_5]
  Transfer Fcn6/1 -> Pow5/1, [ohm_6]
  Saturation/1 -> [ohm2_1]
  Saturation12/1 -> [ohm2_2]
  Saturation13/1 -> [ohm2_3]
  Saturation14/1 -> [ohm2_4]
  Saturation15/1 -> [ohm2_5]
  Saturation16/1 -> [ohm2_6]
  Pow/1 -> Ω2_1/1
  Pow1/1 -> Ω2_2/1
  Pow2/1 -> Ω2_3/1
  Pow3/1 -> Ω2_4/1
  Pow4/1 -> Ω2_5/1
  Pow5/1 -> Ω2_6/1

== system control_UAV/Subsystem4 ==
  z : Inport
  zd : Inport  Port=2
  zp : Inport  Port=3
  Constant : Constant  Value=Thover
  Gain : Gain  Gain=kdz
  Gain1 : Gain  Gain=m
  Gain3 : Gain  Gain=kiz
  Gain5 : Gain  Gain=kpz
  Integrator6 : Integrator
  Sum : Sum  Inputs=|+-
  Sum1 : Sum  Inputs=++-
  Sum2 : Sum  Inputs=|++
  u1 : Outport
  ez : Outport  Port=2
  wires:
  Gain5/1 -> Sum1/1
  z/1 -> Sum/2
  Integrator6/1 -> Sum1/2
  Gain/1 -> Sum1/3
  Gain3/1 -> Integrator6/1
  Sum/1 -> ez/1, Gain5/1, Gain3/1
  zd/1 -> Sum/1
  zp/1 -> Gain/1
  Sum1/1 -> Gain1/1
  Gain1/1 -> Sum2/1
  Sum2/1 -> u1/1
  Constant/1 -> Sum2/2

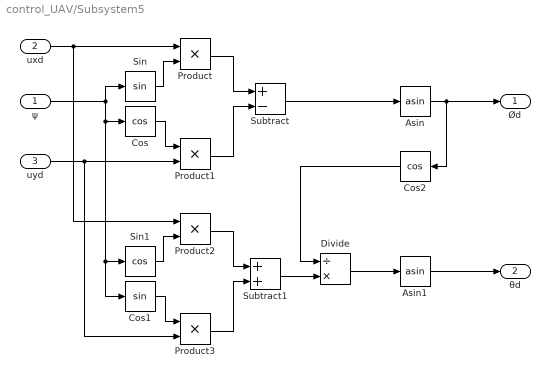
== system control_UAV/Subsystem5 ==
  ψ : Inport
  uxd : Inport  Port=2
  uyd : Inport  Port=3
  Asin : Trigonometry  Operator=asin
  Asin1 : Trigonometry  Operator=asin
  Cos : Trigonometry  Operator=cos
  Cos1 : Trigonometry
  Cos2 : Trigonometry  Operator=cos
  Divide : Product  Inputs=/*
  Product{,1..3} (4 alike) : Product
  Sin : Trigonometry
  Sin1 : Trigonometry  Operator=cos
  Subtract : Sum  Inputs=+-
  Subtract1 : Sum
  Ød : Outport
  θd : Outport  Port=2
  wires:
  ψ/1 -> Sin/1, Cos1/1, Sin1/1, Cos/1
  Sin/1 -> Product/2
  Cos/1 -> Product1/1
  Product/1 -> Subtract/1
  Product1/1 -> Subtract/2
  Asin/1 -> Ød/1, Cos2/1
  Product3/1 -> Subtract1/2
  Product2/1 -> Subtract1/1
  Cos1/1 -> Product3/1
  uyd/1 -> Product3/2, Product1/2
  uxd/1 -> Product/1, Product2/1
  Sin1/1 -> Product2/2
  Subtract1/1 -> Divide/2
  Cos2/1 -> Divide/1
  Asin1/1 -> θd/1
  Subtract/1 -> Asin/1
  Divide/1 -> Asin1/1

== system control_UAV/Subsystem6 ==
  x : Inport
  xd : Inport  Port=2
  xp : Inport  Port=3
  Gain : Gain  Gain=kdx
  Gain3 : Gain  Gain=kix
  Gain5 : Gain  Gain=kpx
  Integrator6 : Integrator
  Sum : Sum  Inputs=|+-
  Sum1 : Sum  Inputs=++-
  uxd : Outport
  ex : Outport  Port=2
  wires:
  xd/1 -> Sum/1
  Sum/1 -> Gain3/1, ex/1, Gain5/1
  Gain3/1 -> Integrator6/1
  Sum1/1 -> uxd/1
  Gain/1 -> Sum1/3
  Integrator6/1 -> Sum1/2
  x/1 -> Sum/2
  Gain5/1 -> Sum1/1
  xp/1 -> Gain/1

== system control_UAV/Subsystem7 ==
  ψ : Inport
  ψd : Inport  Port=2
  ψp : Inport  Port=3
  Gain13 : Gain  Gain=kdpsi
  Gain15 : Gain  Gain=kipsi
  Gain16 : Gain  Gain=kppsi
  Integrator3 : Integrator
  Sum6 : Sum  Inputs=|+-
  Sum7 : Sum  Inputs=++-
  u4 : Outport
  eψ : Outport  Port=2
  wires:
  ψp/1 -> Gain13/1
  ψ/1 -> Sum6/2
  Gain15/1 -> Integrator3/1
  Gain16/1 -> Sum7/1
  Integrator3/1 -> Sum7/2
  Gain13/1 -> Sum7/3
  Sum7/1 -> u4/1
  Sum6/1 -> Gain15/1, eψ/1, Gain16/1
  ψd/1 -> Sum6/1

== system control_UAV/Subsystem8 ==
  y : Inport
  yd : Inport  Port=2
  yp : Inport  Port=3
  Gain : Gain  Gain=kdy
  Gain3 : Gain  Gain=kiy
  Gain5 : Gain  Gain=kpy
  Integrator6 : Integrator
  Sum : Sum  Inputs=|+-
  Sum1 : Sum  Inputs=++-
  uyd : Outport
  ey : Outport  Port=2
  wires:
  yd/1 -> Sum/1
  Sum/1 -> Gain3/1, ey/1, Gain5/1
  Gain3/1 -> Integrator6/1
  Sum1/1 -> uyd/1
  Gain/1 -> Sum1/3
  Integrator6/1 -> Sum1/2
  y/1 -> Sum/2
  Gain5/1 -> Sum1/1
  yp/1 -> Gain/1

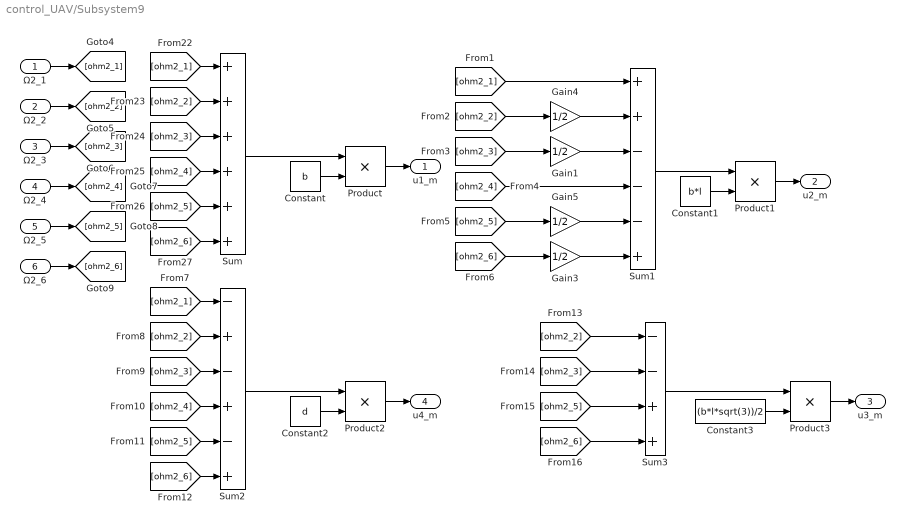
== system control_UAV/Subsystem9 ==
  Ω2_1 : Inport
  Ω2_2 : Inport  Port=2
  Ω2_3 : Inport  Port=3
  Ω2_4 : Inport  Port=4
  Ω2_5 : Inport  Port=5
  Ω2_6 : Inport  Port=6
  Constant : Constant  Value=b
  Constant1 : Constant  Value=b*l
  Constant2 : Constant  Value=d
  Constant3 : Constant  Value=(b*l*sqrt(3))/2
  Gain{1,3..5} (4 alike) : Gain  Gain=1/2
  Product{,1..3} (4 alike) : Product
  Sum : Sum  Inputs=++++++
  Sum1 : Sum  Inputs=++---+
  Sum2 : Sum  Inputs=-+-+-+
  Sum3 : Sum  Inputs=--++
  u1_m : Outport
  u2_m : Outport  Port=2
  u3_m : Outport  Port=3
  u4_m : Outport  Port=4
  wires:
  Sum/1 -> Product/1
  Constant/1 -> Product/2
  Product/1 -> u1_m/1
  Ω2_1/1 -> [ohm2_1]
  Ω2_2/1 -> [ohm2_2]
  Ω2_3/1 -> [ohm2_3]
  Ω2_4/1 -> [ohm2_4]
  Ω2_5/1 -> [ohm2_5]
  Ω2_6/1 -> [ohm2_6]
  [ohm2_1] -> Sum/1
  [ohm2_2] -> Sum/2
  [ohm2_3] -> Sum/3
  [ohm2_4] -> Sum/4
  [ohm2_5] -> Sum/5
  [ohm2_6] -> Sum/6
  [ohm2_2] -> Gain4/1
  Constant1/1 -> Product1/2
  [ohm2_5] -> Gain5/1
  Product1/1 -> u2_m/1
  [ohm2_3] -> Gain1/1
  [ohm2_6] -> Gain3/1
  Sum1/1 -> Product1/1
  [ohm2_1] -> Sum1/1
  Gain1/1 -> Sum1/3
  [ohm2_4] -> Sum1/4
  Gain3/1 -> Sum1/6
  [ohm2_2] -> Sum2/2
  Constant2/1 -> Product2/2
  [ohm2_5] -> Sum2/5
  [ohm2_1] -> Sum2/1
  Product2/1 -> u4_m/1
  [ohm2_3] -> Sum2/3
  [ohm2_6] -> Sum2/6
  [ohm2_4] -> Sum2/4
  Sum2/1 -> Product2/1
  [ohm2_2] -> Sum3/1
  [ohm2_3] -> Sum3/2
  [ohm2_5] -> Sum3/3
  [ohm2_6] -> Sum3/4
  Sum3/1 -> Product3/1
  Product3/1 -> u3_m/1
  Constant3/1 -> Product3/2
  Gain4/1 -> Sum1/2
  Gain5/1 -> Sum1/5

== system control_UAV/Translation axis "X" ==
  ux : Inport
  u1 : Inport  Port=2
  FDx : Inport  Port=3
  Constant : Constant  Value=kftx/m
  Gain1 : Gain  Gain=1/m
  Gain13 : Gain  Gain=1/m
  Integrator : Integrator
  Integrator7 : Integrator
  Product : Product
  Product9 : Product
  Sum : Sum  Inputs=|-++
  xpp : Outport
  xp : Outport  Port=2
  x : Outport  Port=3
  wires:
  Integrator/1 -> xp/1, Product/1, Integrator7/1  "xp"
  Constant/1 -> Product/2
  Product/1 -> Sum/1
  Sum/1 -> xpp/1, Integrator/1  "xpp"
  Integrator7/1 -> x/1  "x"
  ux/1 -> Product9/2
  u1/1 -> Product9/1
  Product9/1 -> Gain13/1
  Gain13/1 -> Sum/2
  FDx/1 -> Gain1/1
  Gain1/1 -> Sum/3

== system control_UAV/Translation axis "Y" ==
  u1 : Inport
  uy : Inport  Port=2
  FDy : Inport  Port=3
  Constant : Constant  Value=kfty/m
  Gain1 : Gain  Gain=1/m
  Gain19 : Gain  Gain=1/m
  Integrator8 : Integrator
  Integrator9 : Integrator
  Product10 : Product
  Product11 : Product
  Sum4 : Sum  Inputs=|-++
  ypp : Outport
  yp : Outport  Port=2
  y : Outport  Port=3
  wires:
  Sum4/1 -> ypp/1, Integrator8/1  "ypp"
  Product10/1 -> Sum4/1
  Constant/1 -> Product10/2
  Integrator8/1 -> Product10/1, yp/1, Integrator9/1  "yp"
  Integrator9/1 -> y/1  "y"
  u1/1 -> Product11/1
  uy/1 -> Product11/2
  Product11/1 -> Gain19/1
  Gain19/1 -> Sum4/2
  FDy/1 -> Gain1/1
  Gain1/1 -> Sum4/3

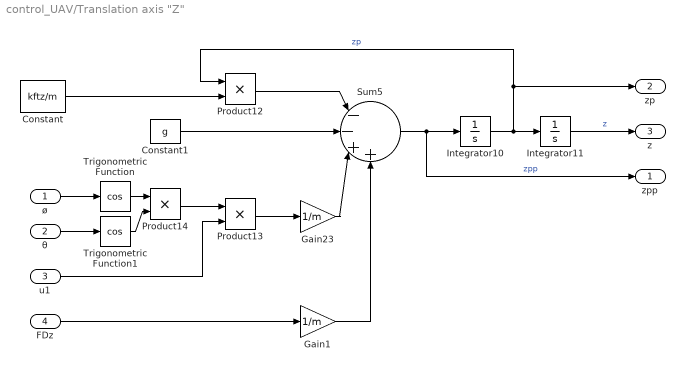
== system control_UAV/Translation axis "Z" ==
  ø : Inport
  θ : Inport  Port=2
  u1 : Inport  Port=3
  FDz : Inport  Port=4
  Constant : Constant  Value=kftz/m
  Constant1 : Constant  Value=g
  Gain1 : Gain  Gain=1/m
  Gain23 : Gain  Gain=1/m
  Integrator10 : Integrator
  Integrator11 : Integrator
  Product12 : Product
  Product13 : Product
  Product14 : Product
  Sum5 : Sum  Inputs=|--++
  Trigonometric Function : Trigonometry  Operator=cos
  Trigonometric Function1 : Trigonometry  Operator=cos
  zpp : Outport
  zp : Outport  Port=2
  z : Outport  Port=3
  wires:
  Trigonometric Function1/1 -> Product14/2
  Constant1/1 -> Sum5/2
  Sum5/1 -> zpp/1, Integrator10/1  "zpp"
  Integrator10/1 -> Product12/1, zp/1, Integrator11/1  "zp"
  Constant/1 -> Product12/2
  Trigonometric Function/1 -> Product14/1
  Product12/1 -> Sum5/1
  Integrator11/1 -> z/1  "z"
  u1/1 -> Product13/2
  ø/1 -> Trigonometric Function/1
  θ/1 -> Trigonometric Function1/1
  Product14/1 -> Product13/1
  Product13/1 -> Gain23/1
  Gain23/1 -> Sum5/3
  FDz/1 -> Gain1/1
  Gain1/1 -> Sum5/4

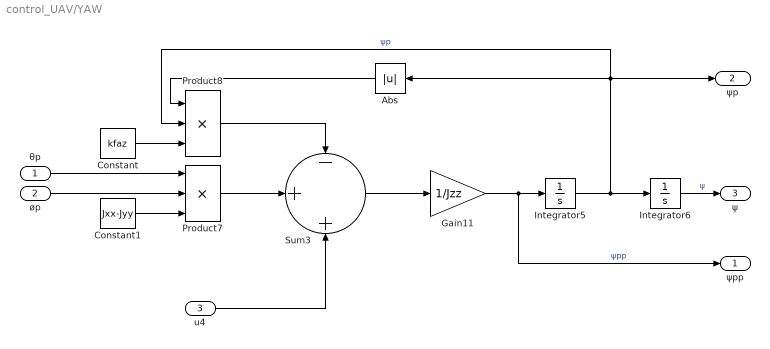
== system control_UAV/YAW ==
  θp : Inport
  øp : Inport  Port=2
  u4 : Inport  Port=3
  Abs : Abs  SaturateOnIntegerOverflow=off
  Constant : Constant  Value=kfaz
  Constant1 : Constant  Value=Jxx-Jyy
  Gain11 : Gain  Gain=1/Jzz
  Integrator5 : Integrator
  Integrator6 : Integrator
  Product7 : Product  Inputs=3
  Product8 : Product  Inputs=3
  Sum3 : Sum  Inputs=-++
  ψpp : Outport
  ψp : Outport  Port=2
  ψ : Outport  Port=3
  wires:
  Product8/1 -> Sum3/1
  Constant/1 -> Product8/3
  Product7/1 -> Sum3/2
  Sum3/1 -> Gain11/1
  Integrator5/1 -> ψp/1, Abs/1, Product8/2, Integrator6/1  "ψp"
  Gain11/1 -> ψpp/1, Integrator5/1  "ψpp"
  Constant1/1 -> Product7/3
  θp/1 -> Product7/1
  u4/1 -> Sum3/3
  øp/1 -> Product7/2
  Integrator6/1 -> ψ/1  "ψ"
  Abs/1 -> Product8/1

== system control_UAV/normalization ==
  x : Inport
  y : Inport  Port=2
  z : Inport  Port=3
  Constant : Constant  Value=chen_center_z
  Gain : Gain  Gain=1/chen_scale_x
  Gain1 : Gain  Gain=1/chen_scale_y
  Gain2 : Gain  Gain=1/chen_scale_z
  Saturation : Saturate  UpperLimit=1  LowerLimit=-1
  Saturation1 : Saturate  UpperLimit=1  LowerLimit=-1
  Saturation2 : Saturate  UpperLimit=1  LowerLimit=-1
  Sum : Sum  Inputs=|+-
  xn : Outport
  yn : Outport  Port=2
  zn : Outport  Port=3
  wires:
  Gain/1 -> Saturation/1
  x/1 -> Gain/1
  Saturation/1 -> xn/1
  Saturation1/1 -> yn/1
  y/1 -> Gain1/1
  Gain1/1 -> Saturation1/1
  Gain2/1 -> Saturation2/1
  Saturation2/1 -> zn/1
  z/1 -> Sum/1
  Sum/1 -> Gain2/1
  Constant/1 -> Sum/2

== system control_UAV/Subsystem3/Subsystem ==
  u1 : Inport
  u2 : Inport  Port=2
  u4 : Inport  Port=3
  Gain : Gain  Gain=1/(6*b*l)
  Gain6 : Gain  Gain=l
  Gain7 : Gain  Gain=2
  Gain8 : Gain  Gain=(b*l)/d
  Sum : Sum  Inputs=++-
  Ω1 : Outport
  wires:
  Gain/1 -> Ω1/1
  u2/1 -> Gain7/1
  Gain8/1 -> Sum/3
  Gain6/1 -> Sum/1
  Sum/1 -> Gain/1
  Gain7/1 -> Sum/2
  u4/1 -> Gain8/1
  u1/1 -> Gain6/1

== system control_UAV/Subsystem3/Subsystem1 ==
  u1 : Inport
  u2 : Inport  Port=2
  u3 : Inport  Port=3
  u4 : Inport  Port=4
  Gain : Gain  Gain=1/(6*b*l)
  Gain1 : Gain  Gain=sqrt(3)
  Gain6 : Gain  Gain=l
  Gain8 : Gain  Gain=(b*l)/d
  Saturation : Saturate  UpperLimit=inf  LowerLimit=0
  Sum : Sum  Inputs=++-+
  Ω2 : Outport
  wires:
  u1/1 -> Gain6/1
  u4/1 -> Gain8/1
  u2/1 -> Sum/2
  Sum/1 -> Gain/1
  Gain6/1 -> Sum/1
  Gain/1 -> Ω2/1
  u3/1 -> Gain1/1
  Gain1/1 -> Sum/3
  Gain8/1 -> Sum/4

== system control_UAV/Subsystem3/Subsystem2 ==
  u1 : Inport
  u2 : Inport  Port=2
  u3 : Inport  Port=3
  u4 : Inport  Port=4
  Gain : Gain  Gain=1/(6*b*l)
  Gain1 : Gain  Gain=sqrt(3)
  Gain6 : Gain  Gain=l
  Gain8 : Gain  Gain=(b*l)/d
  Sum : Sum  Inputs=+---
  Ω3 : Outport
  wires:
  Gain8/1 -> Sum/4
  Gain1/1 -> Sum/3
  u3/1 -> Gain1/1
  Gain/1 -> Ω3/1
  Gain6/1 -> Sum/1
  u2/1 -> Sum/2
  u4/1 -> Gain8/1
  u1/1 -> Gain6/1
  Sum/1 -> Gain/1

== system control_UAV/Subsystem3/Subsystem3 ==
  u1 : Inport
  u2 : Inport  Port=2
  u4 : Inport  Port=3
  Gain : Gain  Gain=1/(6*b*l)
  Gain6 : Gain  Gain=l
  Gain7 : Gain  Gain=2
  Gain8 : Gain  Gain=(b*l)/d
  Sum : Sum  Inputs=+-+
  Ω4 : Outport
  wires:
  u1/1 -> Gain6/1
  u4/1 -> Gain8/1
  Gain7/1 -> Sum/2
  Gain6/1 -> Sum/1
  Gain8/1 -> Sum/3
  u2/1 -> Gain7/1
  Sum/1 -> Gain/1
  Gain/1 -> Ω4/1

== system control_UAV/Subsystem3/Subsystem4 ==
  u1 : Inport
  u2 : Inport  Port=2
  u3 : Inport  Port=3
  u4 : Inport  Port=4
  Gain : Gain  Gain=1/(6*b*l)
  Gain1 : Gain  Gain=sqrt(3)
  Gain6 : Gain  Gain=l
  Gain8 : Gain  Gain=(b*l)/d
  Sum : Sum  Inputs=+-+-
  Ω5 : Outport
  wires:
  u1/1 -> Gain6/1
  u4/1 -> Gain8/1
  Gain6/1 -> Sum/1
  Sum/1 -> Gain/1
  u3/1 -> Gain1/1
  Gain1/1 -> Sum/3
  Gain8/1 -> Sum/4
  u2/1 -> Sum/2
  Gain/1 -> Ω5/1

== system control_UAV/Subsystem3/Subsystem5 ==
  u1 : Inport
  u2 : Inport  Port=2
  u3 : Inport  Port=3
  u4 : Inport  Port=4
  Gain : Gain  Gain=1/(6*b*l)
  Gain1 : Gain  Gain=sqrt(3)
  Gain6 : Gain  Gain=l
  Gain8 : Gain  Gain=(b*l)/d
  Sum : Sum  Inputs=++++
  Ω6 : Outport
  wires:
  u2/1 -> Sum/2
  Gain8/1 -> Sum/4
  Gain1/1 -> Sum/3
  u3/1 -> Gain1/1
  Sum/1 -> Gain/1
  Gain6/1 -> Sum/1
  u4/1 -> Gain8/1
  u1/1 -> Gain6/1
  Gain/1 -> Ω6/1

== matlab function control_UAV/MATLAB Function ==
  data: uxd input; uxd_sat output; uyd input; uyd_sat output
function [uxd_sat, uyd_sat] = saturacion_xy(uxd, uyd)
% Saturación vectorial de las referencias horizontales

% Inclinación máxima permitida
alpha_max = 10*pi/180;

% Magnitud horizontal máxima
rho_max = sin(alpha_max);

% Magnitud solicitada por los controladores X-Y
rho = sqrt(uxd^2 + uyd^2);

% Saturación conservando la dirección
if rho > rho_max
    escala = rho_max / max(rho, 1e-6);

    uxd_sat = escala * uxd;
    uyd_sat = escala * uyd;
else
    uxd_sat = uxd;
    uyd_sat = uyd;
end
end
